simulink model "reference"  (R2023a)
settings: configuration reference "Reference" (kept outside this file)
settings Model: DataDictionary=For_common_config.sldd  Creator=C3020  LastModifiedBy=C9166
settings ConfigSetRef: SourceName=Reference

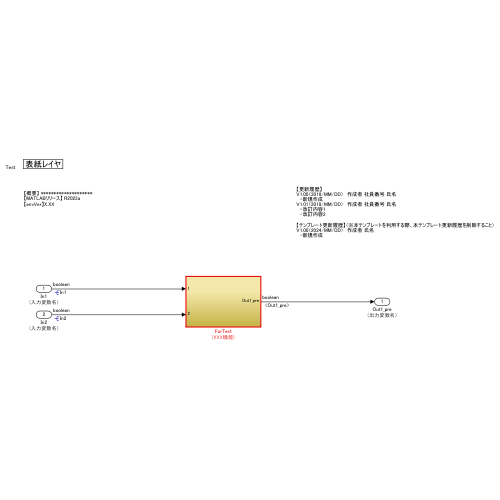
[thumbnail: Simulink's stored preview of the top-level diagram]
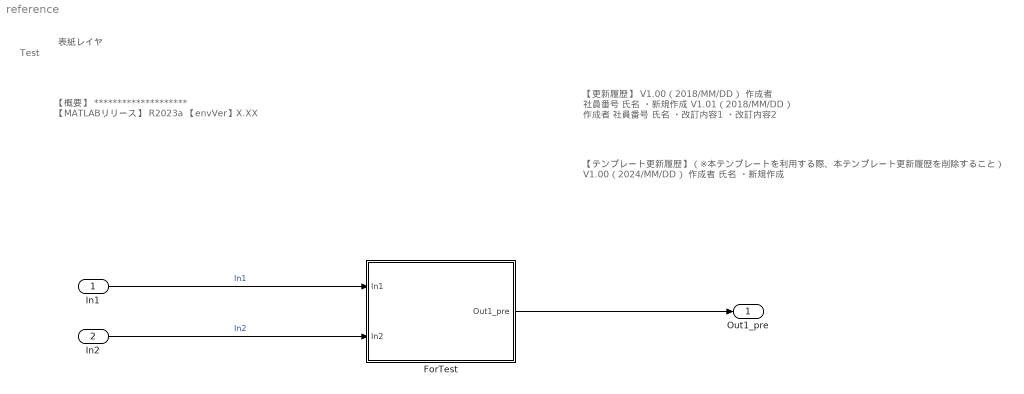
== system reference ==
  note: 表紙レイヤ
  note: 【更新履歴】
      | V1.00（2018/MM/DD）　作成者 社員番号 氏名
      | 　・新規作成
      | V1.01（2018/MM/DD）　作成者 社員番号 氏名
      | 　・改訂内容1
      | 　・改訂内容2
  note: 【テンプレート更新履歴】（※本テンプレートを利用する際、本テンプレート更新履歴を削除すること）
      | V1.00（2024/MM/DD）　作成者 氏名
      | 　・新規作成
  note: 【概要】 ********************
      | 【MATLABリリース】 R2023a
      | 【envVer】X.XX
  note: Test
  In1 : Inport  Description=入力変数名
      settings: AttributesFormatString=(%<Description>)
  In2 : Inport  Description=入力変数名  Port=2
      settings: AttributesFormatString=(%<Description>)
  ForTest : Subsystem  Description=XXX機能  TreatAsAtomicUnit=on
      settings: AttributesFormatString=(%<Description>)
  Out1_pre : Outport  Description=出力変数名
      settings: AttributesFormatString=(%<Description>)
  wires:
  ForTest/1(Out1_pre) -> Out1_pre/1
  In1/1 -> ForTest/1(In1)  "In1"
  In2/1 -> ForTest/2(In2)  "In2"

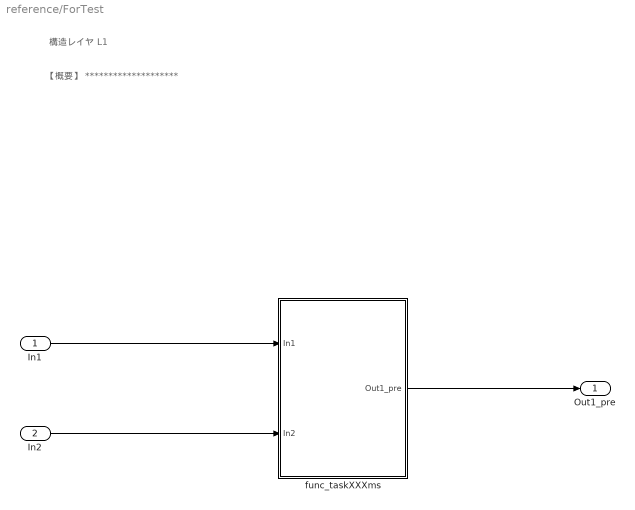
== system reference/ForTest ==
  note: 構造レイヤ L1
  note: 【概要】 ********************
  In1 : Inport  Description=入力変数名
      settings: AttributesFormatString=(%<Description>)
  In2 : Inport  Description=入力変数名  Port=2
      settings: AttributesFormatString=(%<Description>)
  func_taskXXXms : Subsystem  Description=XXX周期タスク  TreatAsAtomicUnit=on
      settings: AttributesFormatString=(%<Description>)
  Out1_pre : Outport  Description=出力変数名
      settings: AttributesFormatString=(%<Description>)
  wires:
  func_taskXXXms/1(Out1_pre) -> Out1_pre/1
  In1/1 -> func_taskXXXms/1(In1)
  In2/1 -> func_taskXXXms/2(In2)

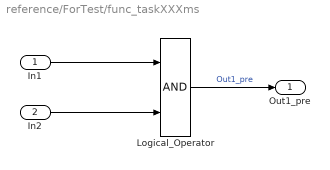
== system reference/ForTest/func_taskXXXms ==
  In1 : Inport  Description=入力変数名
      settings: AttributesFormatString=(%<Description>)
  In2 : Inport  Description=入力変数名  Port=2
      settings: AttributesFormatString=(%<Description>)
  Logical_Operator : Logic  OutDataTypeStr=boolean
  Out1_pre : Outport  Description=出力変数名
      settings: AttributesFormatString=(%<Description>)
  wires:
  Logical_Operator/1 -> Out1_pre/1  "Out1_pre"
  In2/1 -> Logical_Operator/2
  In1/1 -> Logical_Operator/1
